simulink model "Platinum120AV4"  (R2018b)
settings: Solver=FixedStepAuto  StartTime=0.0  StopTime=10.0  RelTol=1e-3
settings Model: Creator=sweat  LastModifiedBy=39926

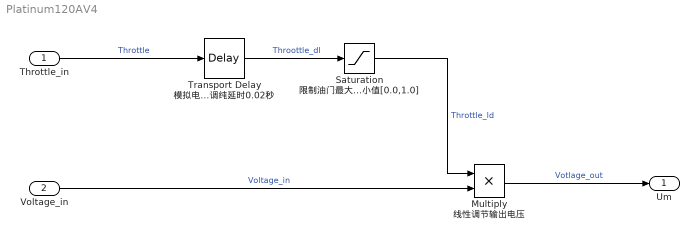
== system Platinum120AV4 ==
  Throttle_in : Inport  PortDimensions=4
  Voltage_in : Inport  Port=2
  Multiply 线性调节输出电压 : Product
  Saturation 限制油门最大最小值[0.0,1.0] : Saturate  UpperLimit=1.0  LowerLimit=0.0
  Transport Delay 模拟电调纯延时0.02秒 : TransportDelay  DelayTime=0.02
  Um : Outport
  wires:
  Throttle_in/1 -> Transport Delay 模拟电调纯延时0.02秒/1  "Throttle"
  Saturation 限制油门最大最小值[0.0,1.0]/1 -> Multiply 线性调节输出电压/1  "Throttle_ld"
  Multiply 线性调节输出电压/1 -> Um/1  "Votlage_out"
  Transport Delay 模拟电调纯延时0.02秒/1 -> Saturation 限制油门最大最小值[0.0,1.0]/1  "Throottle_dl"
  Voltage_in/1 -> Multiply 线性调节输出电压/2  "Voltage_in"
